simulink model "Quiz4_PartD_Simscape"  (R2017b)
settings: Solver=ode14x  StartTime=0.0  StopTime=30  FixedStep=.05  RelTol=1e-3
model workspace (MAT data in the model file):
  Z = 0.01
  w = 3
libraries: fl_lib x6, nesl_utility x3
settings Model: Creator=Harrison  LastModifiedBy=Harrison
settings DataIOCC: SaveFormat=Array

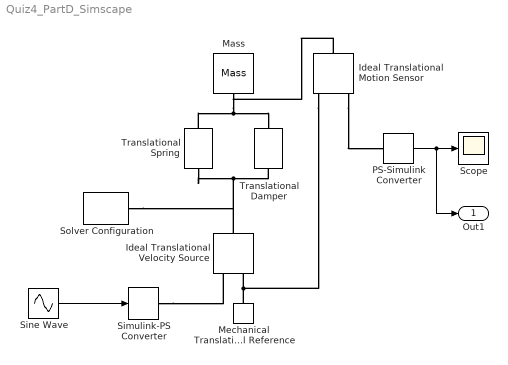
== system Quiz4_PartD_Simscape ==
  Ideal Translational Motion Sensor : fl_lib/Mechanical/Mechanical Sensors/Ideal Translational Motion Sensor  offset=0 m
  Ideal Translational Velocity Source : fl_lib/Mechanical/Mechanical Sources/Ideal Translational Velocity Source
  Mass : fl_lib/Mechanical/Translational Elements/Mass  mass=3000 kg  v_specify=off  v_priority=High  v=0 m/s  v_nominal_specify=off  v_nominal_unit=m/s  v_nominal_value=1  f_specify=off  f_priority=None  f=0 N  f_nominal_specify=off  f_nominal_unit=N  f_nominal_value=1
  Mechanical Translational Reference : fl_lib/Mechanical/Translational Elements/Mechanical Translational Reference
  PS-Simulink Converter : nesl_utility/PS-Simulink Converter  PhysicalDomain=network_engine_domain  SubClassName=ps_output  LeftPortType=input  RightPortType=output  PseudoPeriodic=off  Frequencies=[]  Unit=m  AffineConversion=off
  Scope : Scope
  Simulink-PS Converter : nesl_utility/Simulink-PS Converter  PhysicalDomain=network_engine_domain  SubClassName=ps_input  LeftPortType=input  RightPortType=output  PseudoPeriodic=off  Frequencies=[]  NoiseDistribution=none  NoiseParameters=[]  Unit=m/s  AffineConversion=off  FilteringAndDerivatives=provide  SimscapeFilterOrder=1  InputFilterTimeConstant=0.001  UdotUserProvided=0
  Sine Wave : Sin  Amplitude=Z*w  Frequency=w  Phase=pi/2  SampleTime=0
  Solver Configuration : nesl_utility/Solver Configuration  PhysicalDomain=network_engine_domain  SubClassName=solver  LeftPortType=input  RightPortType=generic  Accelerate=off  Tones=[]  Harmonics=[]  SimulateNoise=off  Profile=off  UseLocalSampling=off  EnableSwitchedLinearOptims=on  FrequencyDomain=off  UseCCode=off  RelTol=0.001  AbsTol=1e-06  MinStep=1e-09  ToWorkspace=off  RevertToSquareIcSolve=off  NumHomotopyIterations=100  PhasorMode=off  PhasorModeNumHarmonics=1  DoDC=off  ResidualTolerance=1e-09  UseLocalSolver=off  LocalSolverChoice=NE_BACKWARD_EULER_ADVANCER  LocalSolverSampleTime=0.001  DoFixedCost=off  MaxNonlinIter=3  MaxModeIter=2  LinearAlgebra=Sparse  DelaysMemoryBudget=1024  AutomaticFiltering=on  FilteringTimeConstant=0.001
  Translational Damper : fl_lib/Mechanical/Translational Elements/Translational Damper  D=2000 N/(m/s)  v_specify=off  v_priority=None  v=0 m/s  v_nominal_specify=off  v_nominal_unit=m/s  v_nominal_value=1  f_specify=off  f_priority=None  f=0 N  f_nominal_specify=off  f_nominal_unit=N  f_nominal_value=1
  Translational Spring : fl_lib/Mechanical/Translational Elements/Translational Spring  spr_rate=50000 N/m  v_specify=off  v_priority=None  v=0 m/s  v_nominal_specify=off  v_nominal_unit=m/s  v_nominal_value=1  f_specify=off  f_priority=None  f=0 N  f_nominal_specify=off  f_nominal_unit=N  f_nominal_value=1  x_specify=off  x_priority=High  x=0 m  x_nominal_specify=off  x_nominal_unit=m  x_nominal_value=1
  Out1 : Outport
  wires:
  PS-Simulink Converter/1 -> Out1/1, Scope/1
  Sine Wave/1 -> Simulink-PS Converter/1
  connections:
  Translational Spring/LConn1 -- Ideal Translational Motion Sensor/LConn1 -- Mass/LConn1 -- Translational Damper/LConn1
  Translational Spring/RConn1 -- Ideal Translational Velocity Source/LConn1 -- Solver Configuration/RConn1 -- Translational Damper/RConn1
  Simulink-PS Converter/RConn1 -- Ideal Translational Velocity Source/RConn1
  Mechanical Translational Reference/LConn1 -- Ideal Translational Motion Sensor/RConn1 -- Ideal Translational Velocity Source/RConn2
  Ideal Translational Motion Sensor/RConn3 -- PS-Simulink Converter/LConn1
